simulink model "TestEncoders"  (R2023b)
settings: Solver=FixedStepAuto  StartTime=0.0  StopTime=inf  RelTol=1e-3  EnableMultiTasking=on
settings Model: ExtModeTrigDuration=2  Creator=Enrique  LastModifiedBy=Enrique
settings OptimizationCC: EnhancedBackFolding=on  PassReuseOutputArgsAs=Individual arguments  ZeroExternalMemoryAtStartup=off  ZeroInternalMemoryAtStartup=off  MaxStackSize=64  OptimizeBlockOrder=speed  DifferentSizesBufferReuse=on  OptimizationCustomize=off  EfficientTunableParamExpr=on
settings DebuggingCC: ParameterTunabilityLossMsg=error
settings HardwareCC: ProdBitPerInt=16  ProdBitPerPointer=16  ProdBitPerSizeT=16  ProdBitPerPtrDiffT=16  ProdLargestAtomicFloat=None  ProdWordSize=8  ProdHWDeviceType=Atmel->AVR  UseEmbeddedCoderFeatures=off  UseSimulinkCoderFeatures=off
settings SFSimCC: MATLABDynamicMemAlloc=off
settings RTWCC: Description=Embedded Coder  SystemTargetFile=ert.tlc  HardwareBoard=Arduino Mega 2560  TemplateMakefile=ert_default_tmf  Toolchain=Arduino AVR  BuildConfiguration=Faster Runs
settings CodeAppCC: ForceParamTrailComments=on  IgnoreCustomStorageClasses=off  OperatorAnnotations=on  SimulinkDataObjDesc=on  SFDataObjDesc=on  MangleLength=10  InsertBlockDesc=on
settings ERTTargetCC: SupportContinuousTime=on  SupportNonInlinedSFcns=on  SupportVariableSizeSignals=on  ExtModeTransport=3  ExtModeStaticAlloc=on  ExtModeAutomaticAllocSize=off  ExtModeStaticAllocSize=2048  ExtModeMexFile=ext_xcp  ExtModeIntrfLevel=Level2 - Open

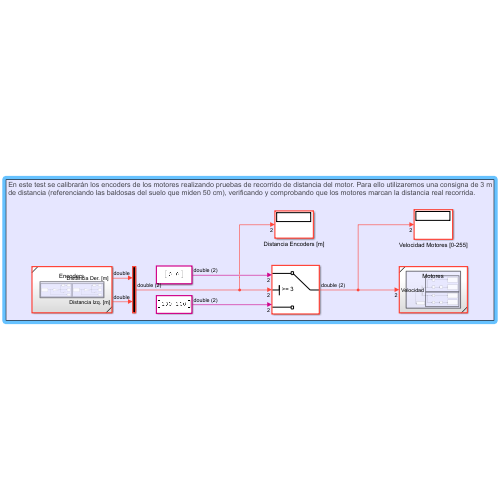
[thumbnail: Simulink's stored preview of the top-level diagram]
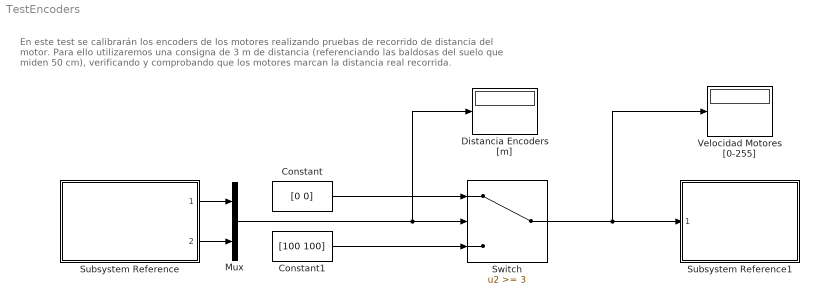
== system TestEncoders ==
  note: En este test se calibrarán los encoders de los motores realizando pruebas de recorrido de distancia del motor. Para ello utilizaremos una consigna de 3 m
      | de distancia (referenciando las baldosas del suelo que miden 50 cm), verificando y comprobando que los motores marcan la distancia real recorrida.
  Constant : Constant  Value=[0 0]
  Constant1 : Constant  Value=[100 100]
  Distancia Encoders [m] : Display
  Mux : Mux  Inputs=2
  Subsystem Reference : Subsystem  ReferencedSubsystem=Encoders
  Subsystem Reference1 : Subsystem  ReferencedSubsystem=Motores
  Switch : Switch  Threshold=3  SaturateOnIntegerOverflow=off  InputSameDT=off
  Velocidad Motores [0-255] : Display
  wires:
  Constant/1 -> Switch/1
  Switch/1 -> Subsystem Reference1/1, Velocidad Motores [0-255]/1
  Constant1/1 -> Switch/3
  Subsystem Reference/2 -> Mux/2
  Subsystem Reference/1 -> Mux/1
  Mux/1 -> Distancia Encoders [m]/1, Switch/2
